simulink model "Discrete_FOC_LSM_v25b"  (R2025b)
settings: Solver=FixedStepDiscrete  StartTime=0.0  StopTime=5  FixedStep=1e-4  MaxStep=0.001  RelTol=1e-3
values from neighbouring files (symbols this model uses):
  airgap_vec = 14.5:1:16.5    [CargarDatosModeloLSM.m]
  Distance_between_EMS = 0.768    [CargarDatosModeloLSM.m]
  force_drag_vec = []    [CargarDatosModeloLSM.m]
  hems_n = 4    [CargarDatosModeloLSM.m]
  init_angle_from_speetec = 4.565126    [CargarDatosModeloLSM.m]
  initial_angle = 0.63    [CargarDatosModeloLSM.m]
  initial_speed = 1    [CargarDatosModeloLSM.m]
  kd = 0.0518    [CargarDatosModeloLSM.m]
  mass = 250    [CargarDatosModeloLSM.m]
  max_voltage = 300    [CargarDatosModeloLSM.m]
  real_airgap = 14.5    [CargarDatosModeloLSM.m]
  speed_drag_vec = 0:5:60    [CargarDatosModeloLSM.m]
  speed_reference_ms = speed_reference/3.6    (= 6.94444444444)    [CargarDatosModeloLSM.m]
  speetec_end = 4 + 2*Distance_between_EMS + 0.5    (= 6.036)    [CargarDatosModeloLSM.m]
  speetec_init = 1 - 0.0925    (= 0.9075)    [CargarDatosModeloLSM.m]
  speetec_offset = 0.174 + 0.116 + 0.0925    (= 0.3825)    [CargarDatosModeloLSM.m]
undefined symbols (not defined in the file or in its folder): angulos, DiscIntNeverNeededParam, frac_polar, fuerza, magnitude, Resistencia
libraries: slpidlib x3, simulink x1
(part 2 of 2)

== matlab function Discrete_FOC_LSM_v25b/MATLAB Function ==
  data: speed_ref_in input; switch_case input; speed_ref_out output; ini_val input
function speed_ref_out = fcn(speed_ref_in,switch_case,ini_val)

persistent rise;
if isempty(rise)
    rise = 0;
end

if switch_case == 1
    rise = switch_case; 
end

speed_ref_out = ini_val; % Only changed when detected speetec
if rise == 1
    speed_ref_out = speed_ref_in;
end

== matlab function Discrete_FOC_LSM_v25b/LSM model/Sensor de Corriente/Sensor corriente W/MATLAB Function1 ==
  data: V input; I output
function I = fcn(V)

I = (V - 2.5)/0.005;

== matlab function Discrete_FOC_LSM_v25b/LSM model/Sensor de Corriente/Sensor corriente W/Sensor ==
  data: I input; V output; Offset input
function V = fcn(I, Offset)

Vcc = 5;                                        %Vcc ??                             La corriente va hasta máximo 5V

if (I > 300)
    I = 300;
end

if (I < -300)
    I = -300;
end


V_ref = Vcc / 2;

V = V_ref + 0.005 * I;

V = V + Offset;                 % Por?


end

== matlab function Discrete_FOC_LSM_v25b/LSM model/Cálculo EMS/Cálculo EMS ==
  settings: updateMethod=DISCRETE
  data: distance_EMS input; speetec_detect input; pos input; numero_EMS output; offset input; pos_value output
function [numero_EMS,pos_value] = fcn(distance_EMS,speetec_detect, pos,offset)

pos_EMS = pos - offset;

persistent speetec_detect_ant
if isempty(speetec_detect_ant)
    speetec_detect_ant = 0;
end

persistent pos_ref
if isempty(pos_ref)
    pos_ref = -1;
end
persistent end_booster
if isempty(end_booster)
    end_booster = 3;
end


if speetec_detect == 1 && speetec_detect_ant == 0
    pos_ref = pos;                 % Is taken as reference the moment the speetec detects the vehicle
end



if pos_ref == -1 || pos_EMS < pos_ref || pos_EMS > (pos_ref + end_booster + 2*distance_EMS)
    numero_EMS = 0;
else
    numero_EMS = 2;

    if pos_EMS >= pos_ref + distance_EMS && pos_EMS <= pos_ref + end_booster + distance_EMS
        numero_EMS = 4;

        if pos_EMS >= pos_ref + 2*distance_EMS && pos_EMS <= pos_ref + end_booster
            numero_EMS = 6;
        end
    end
end
pos_value = pos_ref;
speetec_detect_ant = speetec_detect;

end

== matlab function Discrete_FOC_LSM_v25b/Speetec/Speetec Detection ==
  data: pos input; speetec_detect output; speetec_init input; speetec_end input; pos_for_speetec output
function [speetec_detect,pos_for_speetec] = fcn(pos,speetec_init,speetec_end)

if pos >= speetec_init && pos <= speetec_end         % Begin and end booster
    speetec_detect = 1;
else
    speetec_detect = 0;
end
pos_for_speetec = pos - speetec_init;
end

== matlab function Discrete_FOC_LSM_v25b/LSM model/Cálculo EMS/Subsystem/MATLAB Function ==
  data: in input; out output
function out = fcn(in)

if in < 1
    out = 0;
else
    out = in - 1;
end

== matlab function Discrete_FOC_LSM_v25b/LSM model/Cálculo Dinámica/Cálculo Drag/MATLAB Function3 ==
  data: drag_in input; drag_out output; tiempo input
function drag_out = fcn(drag_in, tiempo)

if tiempo < 1
    drag_out = 0;
else
    drag_out = drag_in;
end



%So doesn't go backward the first moment

== matlab function Discrete_FOC_LSM_v25b/Clark Park/Clarke Transform ==
  data: abc input; AlphaBeta0 output
function AlphaBeta0 = fcn(abc)

M = [1,-1/2,-1/2;0,sqrt(3)/2,-sqrt(3)/2;1/2,1/2,1/2];

AlphaBeta0 = (2/3)*(M*abc);

== matlab function Discrete_FOC_LSM_v25b/Clark Park/Clarke to Park Angle Transform ==
  data: AlphaBeta0 input; dq0 output; ELE_angle input
function dq0 = fcn(AlphaBeta0, ELE_angle)

M = [sin(ELE_angle),-cos(ELE_angle),0; cos(ELE_angle),sin(ELE_angle),0; 0,0,1];

dq0 = M*AlphaBeta0;

== matlab function Discrete_FOC_LSM_v25b/Reverse Park Clark/Inverse Park Transform ==
  data: dq0 input; abc output; ELE_angle input
function abc = fcn(dq0, ELE_angle)

M = [sin(ELE_angle),cos(ELE_angle),1; sin(ELE_angle-(2*pi/3)),cos(ELE_angle-(2*pi/3)),1; sin(ELE_angle+(2*pi/3)),cos(ELE_angle+(2*pi/3)),1];

abc = M*dq0;

end

== matlab function Discrete_FOC_LSM_v25b/LSM model/Phase/Calculate Actual Angle ==
  data: angle_ini input; actual_angle output; angle input
function actual_angle = fcn(angle_ini, angle)
actual_angle = mod(angle_ini + angle,2*pi);
end

== matlab function Discrete_FOC_LSM_v25b/LSM model/Maximun calculation/Frequency and Max Calculator ==
  settings: updateMethod=DISCRETE  sampleTime=1e-4
  data: frecuencia output; value input; Maximo output
function [frecuencia,Maximo]= fcn(value)

%#codegen

% Calculate Frequency and max peak

Ts = 1e-4;

persistent tiempo
if isempty(tiempo)
    tiempo = 0;
end

tiempo = tiempo + Ts;

frecuencia = frecuency_calculator(value, tiempo);
Maximo = maximum_calculator(frecuencia, value, tiempo);

end


% ============================================================
% Calculate Frequency
% ============================================================

function frecuencia = frecuency_calculator(value, tiempo)

persistent signo
if isempty(signo)
   signo = [0 0 0];
end

persistent t_inicio
if isempty(t_inicio)
   t_inicio = [0 0 0];
end

persistent frecuencia_acc
if isempty(frecuencia_acc)
   frecuencia_acc = 1;
end

frecuencia = frecuencia_acc;

for i = 1:3

    if signo(i) == 0

        if value(i) >= 0
            signo(i) = 1;
        else
            signo(i) = 2;
        end

        t_inicio(i) = tiempo;

    end

    if signo(i) == 1

        if value(i) <= 0

            dt = tiempo - t_inicio(i);

            % avoid division by zero
            if dt > 1e-12

                frecuencia = 1 / (2 * dt);
                frecuencia_acc = frecuencia;

            end

            signo(i) = 0;

        end

    end

    if signo(i) == 2

        if value(i) >= 0

            dt = tiempo - t_inicio(i);

            % avoid division by zero
            if dt > 1e-12

                frecuencia = 1 / (2 * dt);
                frecuencia_acc = frecuencia;

            end

            signo(i) = 0;

        end

    end

end

end


% ============================================================
% Calculate Max value
% ============================================================

function Maximo = maximum_calculator(frecuencia, valor, tiempo)

persistent antiguo_maximo
if isempty(antiguo_maximo)
   antiguo_maximo = 0;
end

persistent t_maximo
if isempty(t_maximo)
   t_maximo = 0;
end

maximo = [0 0 0];

frecuencia_abs = abs(frecuencia);

% avoid division by zero
if frecuencia_abs < 1e-12
    frecuencia_abs = 1e-12;
end

periodo = 1 / frecuencia_abs / 3;

for i = 1:3

    if abs(valor(i)) >= antiguo_maximo

        maximo(i) = abs(valor(i));
        antiguo_maximo = abs(valor(i));
        t_maximo = tiempo;

    else

        maximo(i) = antiguo_maximo;

        if tiempo > t_maximo + periodo

            maximo(i) = abs(valor(i));
            antiguo_maximo = abs(valor(i));
            t_maximo = tiempo;

        end

    end

end

Maximo = max(maximo);

end

% function [frecuencia,Maximo]= fcn(value)
%  % Calculate Frequency and max peak
%  Ts = 1e-4;
% 
% persistent tiempo
% if isempty(tiempo)
%     tiempo = 0;
% end
% 
% tiempo = tiempo + Ts;
% 
% frecuencia = frecuency_calculator(value, tiempo);
% Maximo = maximum_calculator(frecuencia, value, tiempo);
% 
% end
% 
% % Calculate Frequency
% function frecuencia = frecuency_calculator(value, tiempo)
%     persistent signo
%     if isempty(signo)
%        signo = [0 0 0]; 
%     end
%     persistent t_inicio
%     if isempty(t_inicio)
%        t_inicio = [0 0 0];
%     end
%     persistent frecuencia_acc
%     if isempty(frecuencia_acc)
%        frecuencia_acc = 1;
%     end
% 
%     frecuencia = frecuencia_acc;
%     for i = 1:3
%         if signo(i) == 0
%             if value(i) >= 0 
%                 signo(i) = 1;
%             else
%                 signo(i) = 2;
%             end
%             t_inicio(i) = tiempo;
%         end
% 
%         if signo(i) == 1
%             if value(i) <= 0
%                 frecuencia = 1 / (2 * (tiempo - t_inicio(i)));
%                 frecuencia_acc = frecuencia;
%                 signo(i) = 0;
%             end
%         end
% 
%         if signo(i) == 2
%             if value(i) >= 0
%                 frecuencia = 1 / (2 * (tiempo - t_inicio(i)));
%                 frecuencia_acc = frecuencia;
%                 signo(i) = 0;
%             end
%         end
%     end
% end
% % Calculate Max value
% function Maximo = maximum_calculator(frecuencia, valor, tiempo)
%     persistent antiguo_maximo
%     if isempty(antiguo_maximo)
%        antiguo_maximo = 0;
%     end
%     persistent t_maximo
%     if isempty(t_maximo)
%        t_maximo = 0;
%     end
% 
%     maximo = [0 0 0];
%     periodo = 1 / abs(frecuencia) / 3;
%     for i = 1:3
%         if abs(valor(i)) >= antiguo_maximo
%             maximo(i) = abs(valor(i));
%             antiguo_maximo = abs(valor(i));
%             t_maximo = tiempo;
%         else
%             maximo(i) = antiguo_maximo;
%             if tiempo > t_maximo + periodo
%                 maximo(i) = abs(valor(i));
%                 antiguo_maximo = abs(valor(i));
%                 t_maximo = tiempo;
%             end
%         end
%     end
%     Maximo = max(maximo);
% end

== matlab function Discrete_FOC_LSM_v25b/LSM model/Sensor de Corriente/Sensor corriente U/Sensor ==
  data: I input; V output; Offset input
function V = fcn(I, Offset)

Vcc = 5;                                        %Vcc ??                             La corriente va hasta máximo 5V

if (I > 300)
    I = 300;
end

if (I < -300)
    I = -300;
end


V_ref = Vcc / 2;

V = V_ref + 0.005 * I;

V = V + Offset;                 % Por?


end

== matlab function Discrete_FOC_LSM_v25b/LSM model/Sensor de Corriente/Sensor corriente U/Discretizado Amplitud ==
  data: valor input; valor_discretizado output; num_valores input; max input; min input
function valor_discretizado = fcn(valor, num_valores, max, min)

if valor > max
    valor_discretizado = max;
    return
end

if valor < min
    valor_discretizado = min;
    return
end


valor_escalon = (max - min)/(num_valores - 1);


i = min;


while (i < max)
    if (i + valor_escalon/2 > valor)
        valor_discretizado = i;
        return
    end

    i = i + valor_escalon;
end


valor_discretizado = max;

end

== matlab function Discrete_FOC_LSM_v25b/LSM model/Sensor de Corriente/Sensor corriente U/MATLAB Function1 ==
  data: V input; I output
function I = fcn(V)

I = (V - 2.5)/0.005;

== matlab function Discrete_FOC_LSM_v25b/LSM model/Sensor de Corriente/Sensor corriente V/Discretizado Amplitud ==
  data: valor input; valor_discretizado output; num_valores input; max input; min input
function valor_discretizado = fcn(valor, num_valores, max, min)

if valor > max
    valor_discretizado = max;
    return
end

if valor < min
    valor_discretizado = min;
    return
end


valor_escalon = (max - min)/(num_valores - 1);


i = min;


while (i < max)
    if (i + valor_escalon/2 > valor)
        valor_discretizado = i;
        return
    end

    i = i + valor_escalon;
end


valor_discretizado = max;

end

== matlab function Discrete_FOC_LSM_v25b/LSM model/Sensor de Corriente/Sensor corriente V/MATLAB Function1 ==
  data: V input; I output
function I = fcn(V)

I = (V - 2.5)/0.005;
